simulink model "CustomerFunction"  (R2024b)
settings: Solver=VariableStepAuto  StartTime=0.0  StopTime=10.0  RelTol=1e-3
settings Model: Creator=ryandavis  LastModifiedBy=ryandavis

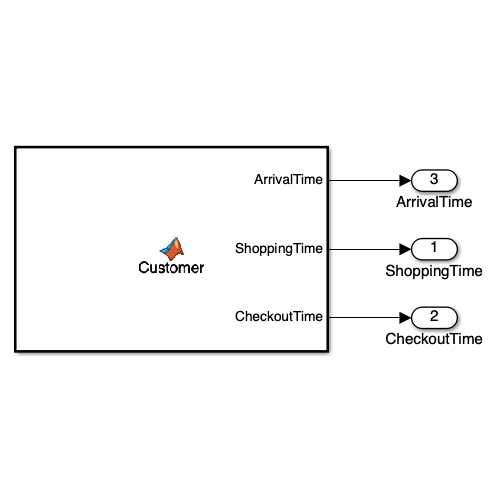
[thumbnail: Simulink's stored preview of the top-level diagram]
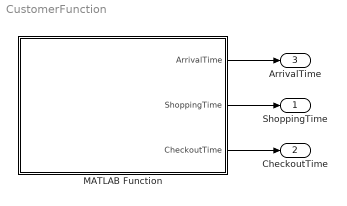
== system CustomerFunction ==
  MATLAB Function : MATLAB Function  TreatAsAtomicUnit=on
  ShoppingTime : Outport
  CheckoutTime : Outport  Port=2
  ArrivalTime : Outport  Port=3
  wires:
  MATLAB Function/2(ShoppingTime) -> ShoppingTime/1
  MATLAB Function/3(CheckoutTime) -> CheckoutTime/1
  MATLAB Function/1(ArrivalTime) -> ArrivalTime/1

== matlab function CustomerFunction/MATLAB Function ==
  data: ArrivalTime output; ShoppingTime output; CheckoutTime output
function [ArrivalTime, ShoppingTime, CheckoutTime] = Customer()
    % Function to generate input variables to match Excel
    ArrivalTime = randi(10);     % Random arrival time between 0-10
    ShoppingTime = randi(7);     % Random shopping time between 1-7
    CheckoutTime = randi(4);     % Random checkout time between 1-4
end
